simulink model "getResponeRobot_Odom"  (R2020a)
settings: Solver=FixedStepAuto  StartTime=0.0  StopTime=28  FixedStep=0.005  RelTol=1e-3
undefined symbols (not defined in the file or in its folder): CR, serial
libraries: instrumentlib x2, simulink x1
settings Model: Creator=dangh  LastModifiedBy=dangh

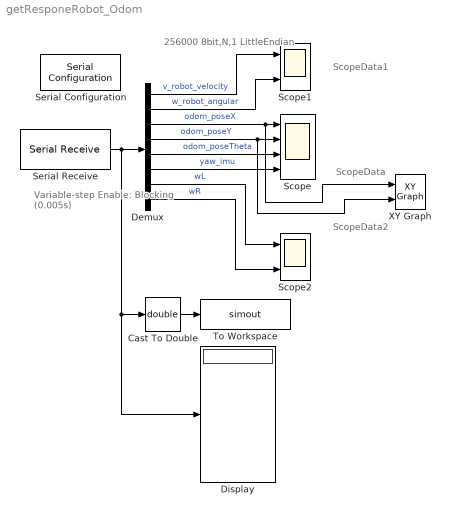
== system getResponeRobot_Odom ==
  note: ScopeData1
  note: ScopeData
  note: 256000
      | 8bit,N,1
      | LittleEndian
  note: Variable-step
      | Enable: Blocking
      | (0.005s)
  note: ScopeData2
  Cast To Double : DataTypeConversion  OutDataTypeStr=double
  Demux : Demux  Outputs=8
  Display : Display
  Scope : Scope  NumInputPorts=4
  Scope1 : Scope  NumInputPorts=2
  Scope2 : Scope  NumInputPorts=2
  Serial Configuration : instrumentlib/Serial Configuration  Priority=-200000  ComPortMenu=COM8  ComPort=COM8  ObjConstructor=serial('COM8');  BaudRate=256000  DataBits=8  Parity=none  StopBits=1  FlowControl=none  Timeout=10  ByteOrder=LittleEndian
  Serial Receive : instrumentlib/Serial Receive  ComPortMenu=COM8  ComPort=COM8  ObjConstructor=serial('COM8');  Terminator=CR ('\r')  DataSize=8  DataType=single  EnableBlockingMode=on  ActionDataUnavailable=Output last received value  CustomValue=0  SampleTime=0.005
  To Workspace : ToWorkspace  VariableName=simout  SaveFormat=Timeseries  SampleTime=-1
  XY Graph : simulink/Sinks/XY Graph  xmin=-1.1  xmax=1.1  ymin=-0.1  ymax=2.1  st=-1
  wires:
  Serial Receive/1 -> Demux/1, Cast To Double/1, Display/1
  Demux/1 -> Scope1/1  "v_robot_velocity"
  Demux/2 -> Scope1/2  "w_robot_angular"
  Demux/3 -> XY Graph/1, Scope/1  "odom_poseX"
  Demux/4 -> XY Graph/2, Scope/2  "odom_poseY"
  Demux/5 -> Scope/3  "odom_poseTheta"
  Demux/6 -> Scope/4  "yaw_imu"
  Demux/7 -> Scope2/1  "wL"
  Demux/8 -> Scope2/2  "wR"
  Cast To Double/1 -> To Workspace/1
